simulink model "PVArrayModel"  (R2015a)
settings: Solver=ode15s  StartTime=0.0  StopTime=12  RelTol=1e-3
libraries: fl_lib x4, nesl_utility x4, elec_lib x1, simulink x1
settings Model: Creator=Lenovo  LastModifiedBy=Lenovo

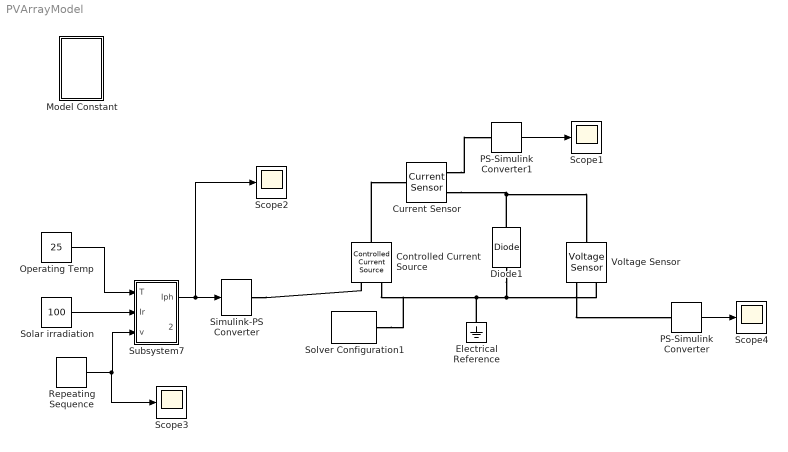
== system PVArrayModel ==
  Controlled Current Source : fl_lib/Electrical/Electrical Sources/Controlled Current Source
  Current Sensor : fl_lib/Electrical/Electrical Sensors/Current Sensor
  Diode1 : elec_lib/Semiconductor Devices/Diode  ModelType=1  Vf=0.6 V  Ron=0.3 Ohm  Goff=1e-8 S  Rz=0.3 Ohm  Vz=50 V  C_PWL=5 pF  prmExp=1  I12=[ 0.0137 0.545 ] A  V12=[ 0.6 0.7 ] V  I1=0.0137 A  V1=0.6 V  RS=0.01 Ohm  IS=1e-12 A  Tmeas=25 C  ec=1  BV=Inf V  C_param=1  CJ0=5 pF  VJ=1 V  Mgrad=0.5  Vvec=[ 0.1 10 100 ] V  Cvec=[ 3.5 1 0.4 ] pF  FC=0.5  Q_param=1  Irrm=-7.15 A  iF=4 A  didt=-750 A/us  trr=115 ns  TT=50 ns  tau=100 ns  T_param=1  IS_T2=1.25e-7 A  I1_T2=0.245 A  V1_T2=0.5 V  Tmeas2=125 C  EG_param=1  EG=1.11 eV  XTI_param=1  XTI=3  dBVdT=0 V/K  Tdevice=25 C  Rth=[ 0 10 ] K/W  thermal_mass_parameterization=1  thermal_mass=[ 0 1 ] J/K  thermal_time_constant=[ 0 10 ] s  thermal_mass_initial_temperatures=[ 25 25 ] C
  Electrical Reference : fl_lib/Electrical/Electrical Elements/Electrical Reference
  Model Constant : Subsystem
  Operating Temp : Constant  Value=25
  PS-Simulink Converter : nesl_utility/PS-Simulink Converter  PhysicalDomain=network_engine_domain  SubClassName=ps_output  LeftPortType=input  RightPortType=output  PseudoPeriodic=off  Frequencies=[]  Unit=V  AffineConversion=off
  PS-Simulink Converter1 : nesl_utility/PS-Simulink Converter  PhysicalDomain=network_engine_domain  SubClassName=ps_output  LeftPortType=input  RightPortType=output  PseudoPeriodic=off  Frequencies=[]  Unit=A  AffineConversion=off
  Repeating Sequence : simulink/Sources/Repeating Sequence  rep_seq_t="[0 1 2 3 4 5  7 8 9 10 11 12]"  rep_seq_y=[0 2 4 6 8 10 12 14 16 18 20 22]
  Scope{1..4} (4 alike) : Scope
      Scope2 settings: SaveName=ScopeData2
      Scope3 settings: SaveName=ScopeData3
  Simulink-PS Converter : nesl_utility/Simulink-PS Converter  PhysicalDomain=network_engine_domain  SubClassName=ps_input  LeftPortType=input  RightPortType=output  PseudoPeriodic=off  Frequencies=[]  NoiseDistribution=none  NoiseParameters=[]  Unit=A  AffineConversion=off  InputFiltering=off  SimscapeFilterOrder=1  InputFilterTimeConstant=0.001  UdotUserProvided=1
  Solar irradiation : Constant  Value=100
  Solver Configuration1 : nesl_utility/Solver Configuration  PhysicalDomain=network_engine_domain  SubClassName=solver  LeftPortType=input  RightPortType=generic  Accelerate=off  Tones=[]  Harmonics=[]  SimulateNoise=off  Profile=off  UseLocalSampling=off  EnableSwitchedLinearOptims=on  FrequencyDomain=off  UseCCode=off  RelTol=0.001  AbsTol=1e-06  MinStep=1e-09  ToWorkspace=off  RevertToSquareIcSolve=off  NumHomotopyIterations=100  DoDC=off  ResidualTolerance=1e-09  UseLocalSolver=off  LocalSolverChoice=NE_BACKWARD_EULER_ADVANCER  LocalSolverSampleTime=0.001  DoFixedCost=off  MaxNonlinIter=3  MaxModeIter=2  LinearAlgebra=Sparse  DelaysMemoryBudget=1024  AutomaticFiltering=on  FilteringTimeConstant=0.001
  Subsystem7 : Subsystem
  Voltage Sensor : fl_lib/Electrical/Electrical Sensors/Voltage Sensor
  wires:
  Solar irradiation/1 -> Subsystem7/2(Ir)
  Operating Temp/1 -> Subsystem7/1("T ")
  PS-Simulink Converter/1 -> Scope4/1
  Subsystem7/1(Iph) -> Scope2/1, Simulink-PS Converter/1
  PS-Simulink Converter1/1 -> Scope1/1
  Repeating Sequence/1 -> Scope3/1, Subsystem7/3("v ")
  connections:
  Diode1/RConn1 -- Current Sensor/RConn2 -- Voltage Sensor/LConn1
  Electrical Reference/LConn1 -- Controlled Current Source/RConn2 -- Solver Configuration1/RConn1 -- Diode1/LConn1 -- Voltage Sensor/RConn2
  Voltage Sensor/RConn1 -- PS-Simulink Converter/LConn1
  Simulink-PS Converter/RConn1 -- Controlled Current Source/RConn1
  Controlled Current Source/LConn1 -- Current Sensor/LConn1
  Current Sensor/RConn1 -- PS-Simulink Converter1/LConn1

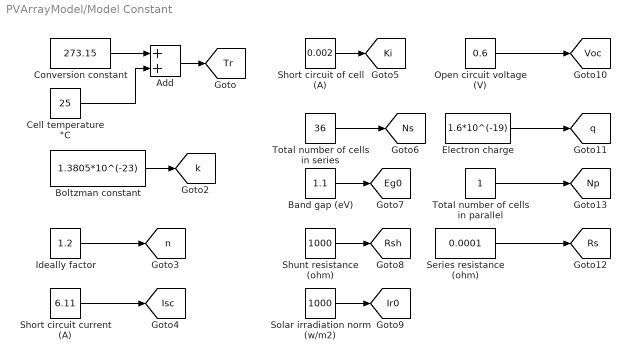
== system PVArrayModel/Model Constant ==
  Add : Sum
  Band gap (eV) : Constant  Value=1.1
  Boltzman constant : Constant  Value=1.3805*10^(-23)
  Cell temperature °C : Constant  Value=25
  Conversion constant : Constant  Value=273.15
  Electron charge : Constant  Value=1.6*10^(-19)
  Ideally factor : Constant  Value=1.2
  Open circuit voltage (V) : Constant  Value=0.6
  Series resistance (ohm) : Constant  Value=0.0001
  Short circuit current (A) : Constant  Value=6.11
  Short circuit of cell (A) : Constant  Value=0.002
  Shunt resistance (ohm) : Constant  Value=1000
  Solar irradiation norm (w/m2) : Constant  Value=1000
  Total number of cells in parallel : Constant
  Total number of cells in series : Constant  Value=36
  tag scope: Eg0=global, Ir0=global, Isc=global, Ki=global, Np=global, Ns=global, Rs=global, Rsh=global, Tr=global, Voc=global, k=global, n=global, q=global
  wires:
  Boltzman constant/1 -> [k]
  Short circuit of cell (A)/1 -> [Ki]
  Band gap (eV)/1 -> [Eg0]
  Shunt resistance (ohm)/1 -> [Rsh]
  Conversion constant/1 -> Add/1
  Ideally factor/1 -> [n]
  Short circuit current (A)/1 -> [Isc]
  Total number of cells in series/1 -> [Ns]
  Add/1 -> [Tr]
  Solar irradiation norm (w/m2)/1 -> [Ir0]
  Open circuit voltage (V)/1 -> [Voc]
  Total number of cells in parallel/1 -> [Np]
  Series resistance (ohm)/1 -> [Rs]
  Electron charge/1 -> [q]
  Cell temperature °C/1 -> Add/2

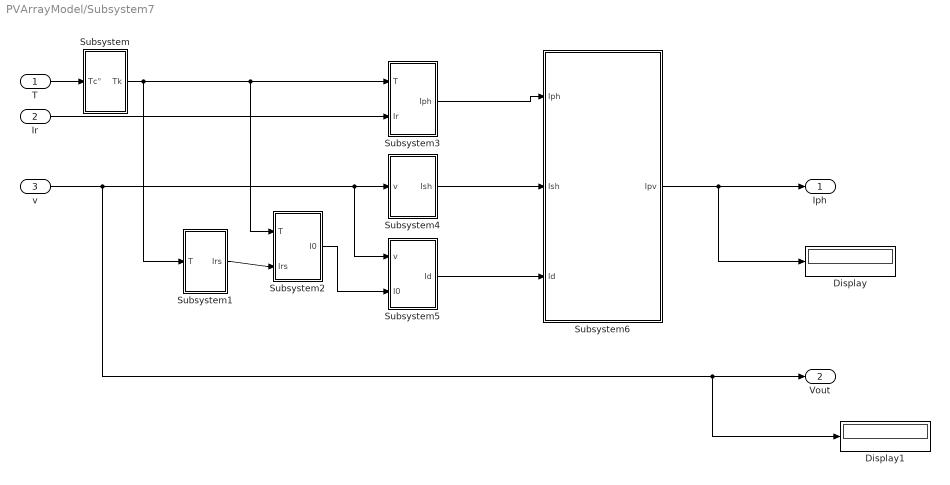
== system PVArrayModel/Subsystem7 ==
  "T " : Inport
  Ir : Inport  Port=2
  "v " : Inport  Port=3
  Display : Display
  Display1 : Display
  Subsystem : Subsystem
  Subsystem1 : Subsystem
  Subsystem2 : Subsystem
  Subsystem3 : Subsystem
  Subsystem4 : Subsystem
  Subsystem5 : Subsystem
  Subsystem6 : Subsystem
  Iph : Outport
  Vout : Outport  Port=2
  wires:
  Subsystem6/1(Ipv) -> Display/1, Iph/1
  "v "/1 -> Display1/1, Vout/1, Subsystem5/1("v "), Subsystem4/1("v ")
  Subsystem3/1(Iph) -> Subsystem6/1("Iph ")
  Subsystem1/1(Irs) -> Subsystem2/2(" Irs")
  Subsystem4/1(Ish) -> Subsystem6/2(Ish)
  Subsystem/1(Tk) -> Subsystem1/1("T "), Subsystem2/1(" T "), Subsystem3/1("T ")
  "T "/1 -> Subsystem/1("Tc° ")
  Subsystem5/1(Id) -> Subsystem6/3(Id)
  Ir/1 -> Subsystem3/2(Ir)
  Subsystem2/1(I0) -> Subsystem5/2(I0)

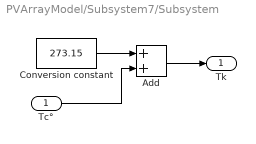
== system PVArrayModel/Subsystem7/Subsystem ==
  "Tc° " : Inport
  Add : Sum
  Conversion constant : Constant  Value=273.15
  Tk : Outport
  wires:
  Conversion constant/1 -> Add/1
  Add/1 -> Tk/1
  "Tc° "/1 -> Add/2

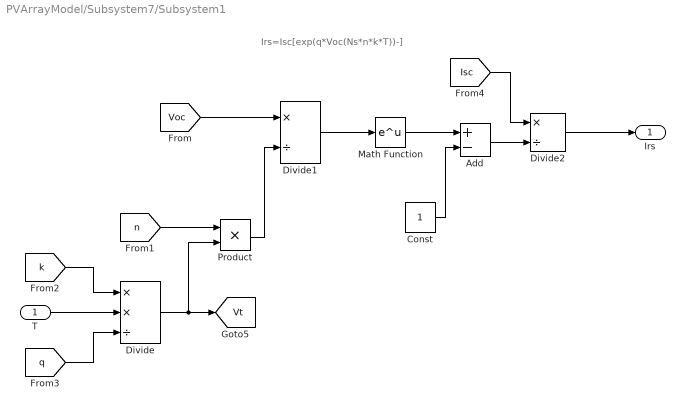
== system PVArrayModel/Subsystem7/Subsystem1 ==
  note: Irs=Isc[exp(q*Voc(Ns*n*k*T))-]
  "T " : Inport
  Add : Sum  Inputs=+-
  Const : Constant
  Divide : Product  Inputs=**/
  Divide1 : Product  Inputs=*/
  Divide2 : Product  Inputs=*/
  Math Function : Math  SaturateOnIntegerOverflow=on
  Product : Product
  Irs : Outport
  tag scope: Vt=global
  wires:
  Const/1 -> Add/2
  [Voc] -> Divide1/1
  [n] -> Product/1
  Divide/1 -> Product/2, [Vt]
  [k] -> Divide/1
  Product/1 -> Divide1/2
  Add/1 -> Divide2/2
  Divide2/1 -> Irs/1
  Math Function/1 -> Add/1
  "T "/1 -> Divide/2
  [Isc] -> Divide2/1
  [q] -> Divide/3
  Divide1/1 -> Math Function/1

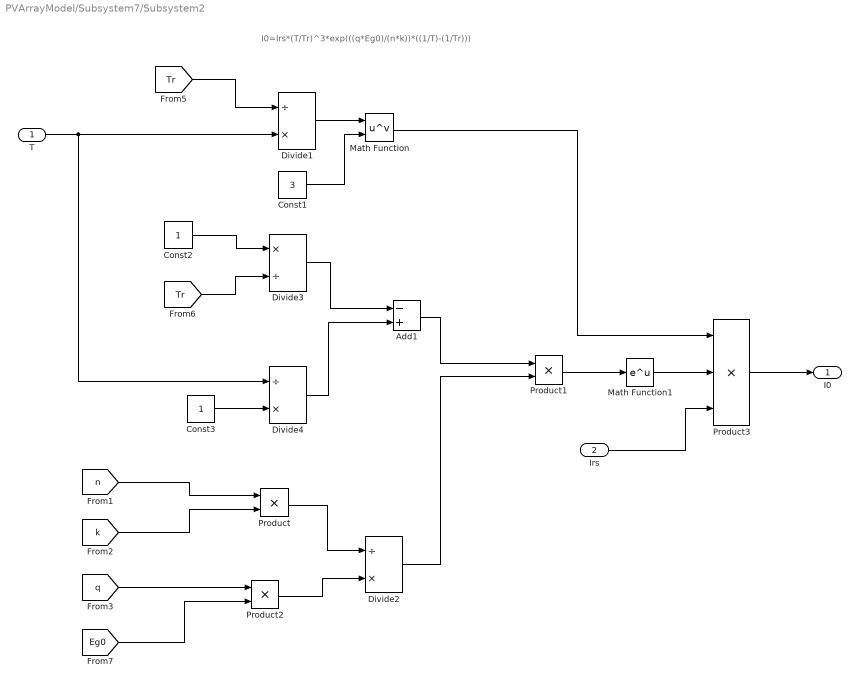
== system PVArrayModel/Subsystem7/Subsystem2 ==
  note: I0=Irs*(T/Tr)^3*exp(((q*Eg0)/(n*k))*((1/T)-(1/Tr)))
  " T " : Inport
  " Irs" : Inport  Port=2
  Add1 : Sum  Inputs=-+
  Const1 : Constant  Value=3
  Const2 : Constant
  Const3 : Constant
  Divide1 : Product  Inputs=/*
  Divide2 : Product  Inputs=/*
  Divide3 : Product  Inputs=*/
  Divide4 : Product  Inputs=/*
  Math Function : Math  Operator=pow  SaturateOnIntegerOverflow=on
  Math Function1 : Math  SaturateOnIntegerOverflow=on
  Product : Product
  Product1 : Product
  Product2 : Product
  Product3 : Product  Inputs=3
  I0 : Outport
  wires:
  [Tr] -> Divide1/1
  [n] -> Product/1
  Divide1/1 -> Math Function/1
  " T "/1 -> Divide4/1, Divide1/2
  Const1/1 -> Math Function/2
  Const2/1 -> Divide3/1
  [Tr] -> Divide3/2
  Divide3/1 -> Add1/1
  Const3/1 -> Divide4/2
  Divide4/1 -> Add1/2
  Add1/1 -> Product1/1
  [k] -> Product/2
  [q] -> Product2/1
  [Eg0] -> Product2/2
  Divide2/1 -> Product1/2
  Product/1 -> Divide2/1
  Product2/1 -> Divide2/2
  Product1/1 -> Math Function1/1
  Math Function/1 -> Product3/1
  Math Function1/1 -> Product3/2
  " Irs"/1 -> Product3/3
  Product3/1 -> I0/1

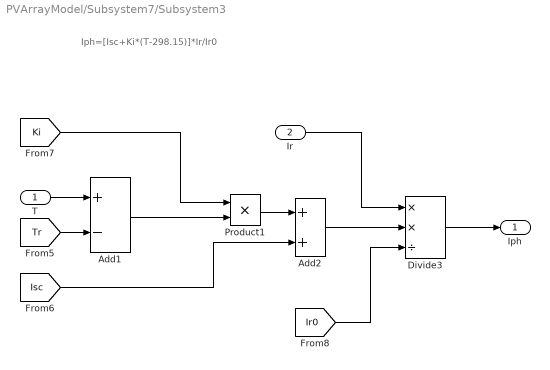
== system PVArrayModel/Subsystem7/Subsystem3 ==
  note: Iph=[Isc+Ki*(T-298.15)]*Ir/Ir0
  "T " : Inport
  Ir : Inport  Port=2
  Add1 : Sum  Inputs=+-
  Add2 : Sum
  Divide3 : Product  Inputs=**/
  Product1 : Product
  Iph : Outport
  wires:
  "T "/1 -> Add1/1
  [Tr] -> Add1/2
  Add1/1 -> Product1/2
  [Ki] -> Product1/1
  Product1/1 -> Add2/1
  [Isc] -> Add2/2
  Add2/1 -> Divide3/2
  Ir/1 -> Divide3/1
  [Ir0] -> Divide3/3
  Divide3/1 -> Iph/1

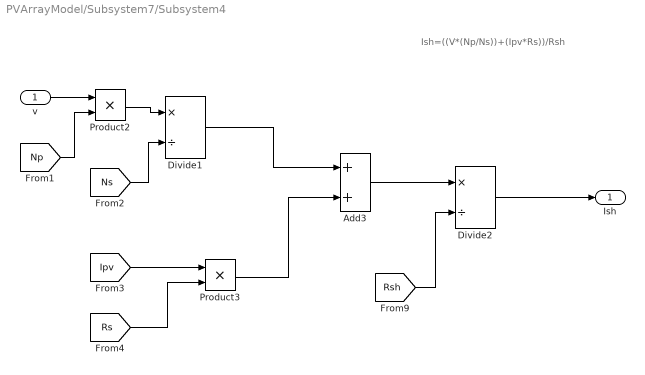
== system PVArrayModel/Subsystem7/Subsystem4 ==
  note: Ish=((V*(Np/Ns))+(Ipv*Rs))/Rsh
  "v " : Inport
  Add3 : Sum
  Divide1 : Product  Inputs=*/
  Divide2 : Product  Inputs=*/
  Product2 : Product
  Product3 : Product
  Ish : Outport
  wires:
  "v "/1 -> Product2/1
  [Np] -> Product2/2
  Product2/1 -> Divide1/1
  [Ns] -> Divide1/2
  [Ipv] -> Product3/1
  [Rs] -> Product3/2
  Divide1/1 -> Add3/1
  Product3/1 -> Add3/2
  Add3/1 -> Divide2/1
  [Rsh] -> Divide2/2
  Divide2/1 -> Ish/1

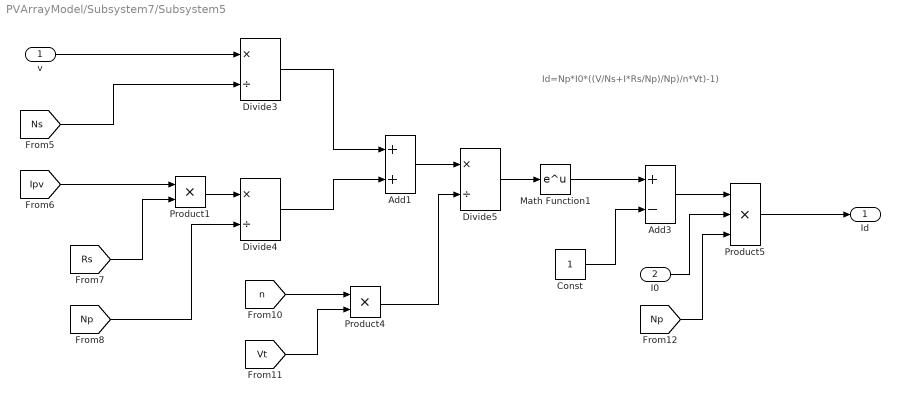
== system PVArrayModel/Subsystem7/Subsystem5 ==
  note: Id=Np*I0*((V/Ns+I*Rs/Np)/Np)/n*Vt)-1)
  "v " : Inport
  I0 : Inport  Port=2
  Add1 : Sum
  Add3 : Sum  Inputs=+-
  Const : Constant
  Divide3 : Product  Inputs=*/
  Divide4 : Product  Inputs=*/
  Divide5 : Product  Inputs=*/
  Math Function1 : Math  SaturateOnIntegerOverflow=on
  Product1 : Product
  Product4 : Product
  Product5 : Product  Inputs=3
  Id : Outport
  wires:
  "v "/1 -> Divide3/1
  [Ns] -> Divide3/2
  [Ipv] -> Product1/1
  [Rs] -> Product1/2
  Product1/1 -> Divide4/1
  [Np] -> Divide4/2
  Divide3/1 -> Add1/1
  Divide4/1 -> Add1/2
  Add1/1 -> Divide5/1
  Divide5/1 -> Math Function1/1
  [n] -> Product4/1
  [Vt] -> Product4/2
  Product4/1 -> Divide5/2
  Math Function1/1 -> Add3/1
  Const/1 -> Add3/2
  Add3/1 -> Product5/1
  [Np] -> Product5/3
  I0/1 -> Product5/2
  Product5/1 -> Id/1

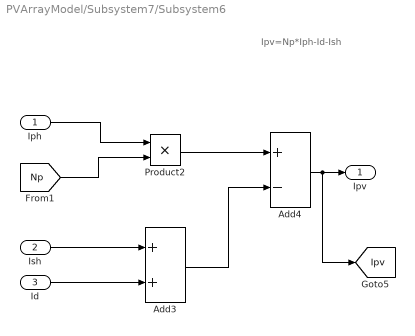
== system PVArrayModel/Subsystem7/Subsystem6 ==
  note: Ipv=Np*Iph-Id-Ish
  "Iph " : Inport
  Ish : Inport  Port=2
  Id : Inport  Port=3
  Add3 : Sum
  Add4 : Sum  Inputs=+-
  Product2 : Product
  Ipv : Outport
  tag scope: Ipv=global
  wires:
  Ish/1 -> Add3/1
  Id/1 -> Add3/2
  "Iph "/1 -> Product2/1
  [Np] -> Product2/2
  Product2/1 -> Add4/1
  Add3/1 -> Add4/2
  Add4/1 -> [Ipv], Ipv/1
